simulink model "nonlinear_model_inverted_pendulum"  (R2024b)
settings: Solver=ode45  StartTime=0.0  StopTime=50  RelTol=1e-6
values from neighbouring files (symbols this model uses):
  b = 0.05    [sim_nonlinear_model_inverted_pendulum.m]
  d = r*2    (= 2)    [plotPendulo.m]    (also in sim_nonlinear_model_inverted_pendulum.m = 0.005; updatePendulo.m)
  dtheta0 = 0    [sim_nonlinear_model_inverted_pendulum.m]
  g = 9.81    [sim_nonlinear_model_inverted_pendulum.m]
  I = 0.099    [sim_nonlinear_model_inverted_pendulum.m]
  Kd1 = 0    [sim_nonlinear_model_inverted_pendulum.m]
  Kd2 = 0    [sim_nonlinear_model_inverted_pendulum.m]
  Ki1 = 0    [sim_nonlinear_model_inverted_pendulum.m]
  Ki2 = 0    [sim_nonlinear_model_inverted_pendulum.m]
  Kp1 = 0    [sim_nonlinear_model_inverted_pendulum.m]
  Kp2 = 0    [sim_nonlinear_model_inverted_pendulum.m]
  l = 40    [plotPendulo.m]    (also in sim_nonlinear_model_inverted_pendulum.m = 0.4; updatePendulo.m)
  M = 2.4    [sim_nonlinear_model_inverted_pendulum.m]
  m = 0.23    [sim_nonlinear_model_inverted_pendulum.m]    (also in unwrap.m = length(p))
  N1 = 100    [sim_nonlinear_model_inverted_pendulum.m]
  N2 = 100    [sim_nonlinear_model_inverted_pendulum.m]
  theta0 = deg2rad(5)    [sim_nonlinear_model_inverted_pendulum.m]
  theta_ref = 0    [sim_nonlinear_model_inverted_pendulum.m]
  v0 = 0    [sim_nonlinear_model_inverted_pendulum.m]
  x0 = 0.2    [sim_nonlinear_model_inverted_pendulum.m]
  x_ref = 0    [sim_nonlinear_model_inverted_pendulum.m]
undefined symbols (not defined in the file or in its folder): magnitude
libraries: slpidlib x2
settings Model: Creator=engma  LastModifiedBy=engma
settings DebuggingCC: AlgebraicLoopMsg=none

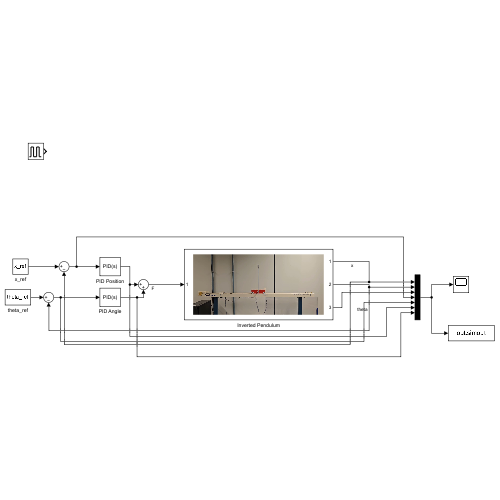
[thumbnail: Simulink's stored preview of the top-level diagram]
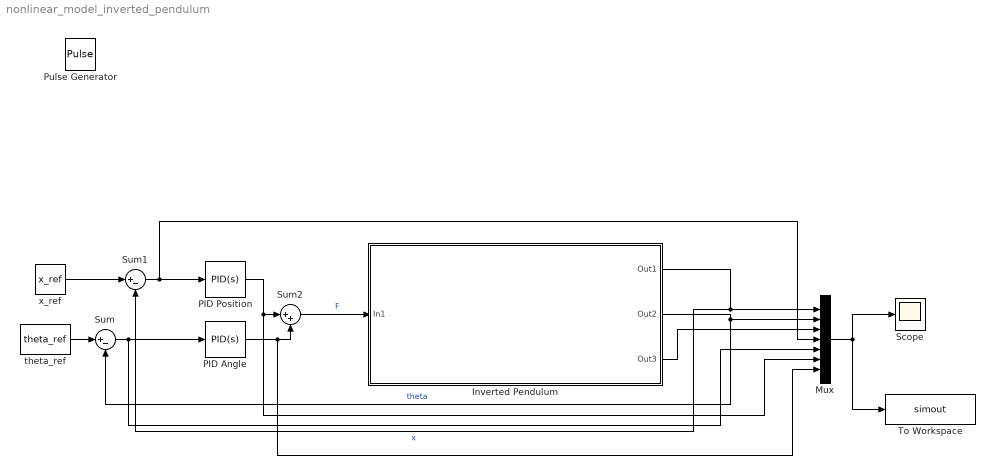
== system nonlinear_model_inverted_pendulum ==
  Inverted Pendulum : Subsystem
      mask Display: image('inverted_pendulum.jpg', [10,10,10,10,100,100]);
  Mux : Mux  Inputs=7
  PID Angle : slpidlib/PID Controller  Controller=PID  Form=Parallel  TimeDomain=Continuous-time  UseExternalTs=off  SampleTime=-1  IntegratorMethod=Forward Euler  FilterMethod=Forward Euler  ControllerParametersSource=internal  P=Kp2  I=Ki2  UseKiTs=off  D=Kd2  UseExternalDerivativeSource=off  N=N2  UseFilter=on  TunerSelectOption=Transfer Function Based (PID Tuner App)  InitialConditionSource=internal  InitialConditionForIntegrator=0  InitialConditionForFilter=0  DifferentiatorICPrevScaledInput=0  ExternalReset=none  TrackingMode=off  Kt=1  LimitOutput=off  SatLimitsSource=internal  UpperSaturationLimit=inf  LowerSaturationLimit=-inf  LinearizeAsGain=on  AntiWindupMode=none  Kb=1  LimitIntegrator=off  UpperIntegratorSaturationLimit=inf  LowerIntegratorSaturationLimit=-inf  POutMin=[]  POutMax=[]  IOutMin=[]  IOutMax=[]  DOutMin=[]  DOutMax=[]  NOutMin=[]  NOutMax=[]  SumOutMin=[]  SumOutMax=[]  SaturationOutMin=[]  SaturationOutMax=[]  PParamMin=[]  PParamMax=[]  IParamMin=[]  IParamMax=[]  DParamMin=[]  DParamMax=[]  NParamMin=[]  NParamMax=[]  KbParamMin=[]  KbParamMax=[]  KtParamMin=[]  KtParamMax=[]  KbOutMin=[]  KbOutMax=[]  KtOutMin=[]  KtOutMax=[]  IntegratorOutMin=[]  IntegratorOutMax=[]  FilterOutMin=[]  FilterOutMax=[]  SumI1OutMin=[]  SumI1OutMax=[]  SumI2OutMin=[]  SumI2OutMax=[]  SumI3OutMin=[]  SumI3OutMax=[]  SumI4OutMin=[]  SumI4OutMax=[]  SumDOutMin=[]  SumDOutMax=[]  DifferentiatorOutMin=[]  DifferentiatorOutMax=[]  FilterDiffOutCoefMin=[]  FilterDiffOutCoefMax=[]  ReciprocalOutMin=[]  ReciprocalOutMax=[]  SumDenOutMin=[]  SumDenOutMax=[]  SumNumOutMin=[]  SumNumOutMax=[]  DivideOutMin=[]  DivideOutMax=[]  UdiffTsProdOutMin=[]  UdiffTsProdOutMax=[]  NTsProdOutMin=[]  NTsProdOutMax=[]  UintegralTsProdOutMin=[]  UintegralTsProdOutMax=[]  UngainTsProdOutMin=[]  UngainTsProdOutMax=[]  ClampingZeroOutDataTypeStr=Inherit: Inherit via back propagation  ClampingZeroOutMin=[]  ClampingZeroOutMax=[]  FilterDenConstantOutDataTypeStr=Inherit: Inherit via back propagation  FilterDenConstantOutMin=[]  FilterDenConstantOutMax=[]  PCopyOutDataTypeStr=Inherit: Inherit via back propagation  PCopyOutMin=[]  PCopyOutMax=[]  NCopyOutDataTypeStr=Inherit: Inherit via back propagation  NCopyOutMin=[]  NCopyOutMax=[]  IntegratorContinuousStateAttributes=''  IntegratorStateMustResolveToSignalObject=off  IntegratorRTWStateStorageClass=Auto  FilterContinuousStateAttributes=''  FilterStateMustResolveToSignalObject=off  FilterRTWStateStorageClass=Auto  ParallelPVariant=InternalParameters  IdealPVariant=Disabled  IVariant=InternalParameters  DVariant=InternalParameters  IntegratorVariant=Continuous  SatVariant=Disabled  AWVariant=Passthrough  PCopyVariant=Disabled  TRVariant=Disabled  FdbkBlocksVariant=Forward  IdealPFdbkVariant=Disabled  SatFdbkVariant=Disabled  DerivativeFilterVariant=ContFilter  NVariant=InternalParameters  NCopyVariant=Disabled  FilterICVariant=InternalICsFilter  IntegratorICVariant=InternalICs  ExternalResetVariant=Disabled  TRSumVariant=Passthrough  SumFdbkVariant=Disabled  SumVariant=Sum_PID  TsampFilterVariant=InternalTs  TsampNgainVariant=Passthrough  TsampIntegralVariant=Disabled_SignalSpec  ExternalSaturationOutDataTypeStr=Inherit: Same as second input  DerivativeSourceVariant=ErrorSignal  PreIntVariant=InternalPreInt
  PID Position : slpidlib/PID Controller  Controller=PID  Form=Parallel  TimeDomain=Continuous-time  UseExternalTs=off  SampleTime=-1  IntegratorMethod=Forward Euler  FilterMethod=Forward Euler  ControllerParametersSource=internal  P=Kp1  I=Ki1  UseKiTs=off  D=Kd1  UseExternalDerivativeSource=off  N=N1  UseFilter=on  TunerSelectOption=Transfer Function Based (PID Tuner App)  InitialConditionSource=internal  InitialConditionForIntegrator=0  InitialConditionForFilter=0  DifferentiatorICPrevScaledInput=0  ExternalReset=none  TrackingMode=off  Kt=1  LimitOutput=off  SatLimitsSource=internal  UpperSaturationLimit=inf  LowerSaturationLimit=-inf  LinearizeAsGain=on  AntiWindupMode=none  Kb=1  LimitIntegrator=off  UpperIntegratorSaturationLimit=inf  LowerIntegratorSaturationLimit=-inf  POutMin=[]  POutMax=[]  IOutMin=[]  IOutMax=[]  DOutMin=[]  DOutMax=[]  NOutMin=[]  NOutMax=[]  SumOutMin=[]  SumOutMax=[]  SaturationOutMin=[]  SaturationOutMax=[]  PParamMin=[]  PParamMax=[]  IParamMin=[]  IParamMax=[]  DParamMin=[]  DParamMax=[]  NParamMin=[]  NParamMax=[]  KbParamMin=[]  KbParamMax=[]  KtParamMin=[]  KtParamMax=[]  KbOutMin=[]  KbOutMax=[]  KtOutMin=[]  KtOutMax=[]  IntegratorOutMin=[]  IntegratorOutMax=[]  FilterOutMin=[]  FilterOutMax=[]  SumI1OutMin=[]  SumI1OutMax=[]  SumI2OutMin=[]  SumI2OutMax=[]  SumI3OutMin=[]  SumI3OutMax=[]  SumI4OutMin=[]  SumI4OutMax=[]  SumDOutMin=[]  SumDOutMax=[]  DifferentiatorOutMin=[]  DifferentiatorOutMax=[]  FilterDiffOutCoefMin=[]  FilterDiffOutCoefMax=[]  ReciprocalOutMin=[]  ReciprocalOutMax=[]  SumDenOutMin=[]  SumDenOutMax=[]  SumNumOutMin=[]  SumNumOutMax=[]  DivideOutMin=[]  DivideOutMax=[]  UdiffTsProdOutMin=[]  UdiffTsProdOutMax=[]  NTsProdOutMin=[]  NTsProdOutMax=[]  UintegralTsProdOutMin=[]  UintegralTsProdOutMax=[]  UngainTsProdOutMin=[]  UngainTsProdOutMax=[]  ClampingZeroOutDataTypeStr=Inherit: Inherit via back propagation  ClampingZeroOutMin=[]  ClampingZeroOutMax=[]  FilterDenConstantOutDataTypeStr=Inherit: Inherit via back propagation  FilterDenConstantOutMin=[]  FilterDenConstantOutMax=[]  PCopyOutDataTypeStr=Inherit: Inherit via back propagation  PCopyOutMin=[]  PCopyOutMax=[]  NCopyOutDataTypeStr=Inherit: Inherit via back propagation  NCopyOutMin=[]  NCopyOutMax=[]  IntegratorContinuousStateAttributes=''  IntegratorStateMustResolveToSignalObject=off  IntegratorRTWStateStorageClass=Auto  FilterContinuousStateAttributes=''  FilterStateMustResolveToSignalObject=off  FilterRTWStateStorageClass=Auto  ParallelPVariant=InternalParameters  IdealPVariant=Disabled  IVariant=InternalParameters  DVariant=InternalParameters  IntegratorVariant=Continuous  SatVariant=Disabled  AWVariant=Passthrough  PCopyVariant=Disabled  TRVariant=Disabled  FdbkBlocksVariant=Forward  IdealPFdbkVariant=Disabled  SatFdbkVariant=Disabled  DerivativeFilterVariant=ContFilter  NVariant=InternalParameters  NCopyVariant=Disabled  FilterICVariant=InternalICsFilter  IntegratorICVariant=InternalICs  ExternalResetVariant=Disabled  TRSumVariant=Passthrough  SumFdbkVariant=Disabled  SumVariant=Sum_PID  TsampFilterVariant=InternalTs  TsampNgainVariant=Passthrough  TsampIntegralVariant=Disabled_SignalSpec  ExternalSaturationOutDataTypeStr=Inherit: Same as second input  DerivativeSourceVariant=ErrorSignal  PreIntVariant=InternalPreInt
  Pulse Generator : DiscretePulseGenerator  PulseType=Time based  Period=100  PulseWidth=5
  Scope : Scope
  Sum : Sum  Inputs=|+-
  Sum1 : Sum  Inputs=|+-
  Sum2 : Sum  Inputs=|++
  To Workspace : ToWorkspace  VariableName=simout  SaveFormat=Structure With Time  SampleTime=-1
  theta_ref : Constant  Value=theta_ref
  x_ref : Constant  Value=x_ref
  wires:
  Inverted Pendulum/1(Out1) -> Mux/1, Sum1/2  "x"
  Inverted Pendulum/2(Out2) -> Sum/2, Mux/2  "theta"
  Mux/1 -> Scope/1, To Workspace/1
  theta_ref/1 -> Sum/1
  x_ref/1 -> Sum1/1
  Sum/1 -> Mux/5, PID Angle/1
  Sum2/1 -> Inverted Pendulum/1(In1)  "F"
  Inverted Pendulum/3(Out3) -> Mux/3
  Sum1/1 -> PID Position/1, Mux/4
  PID Angle/1 -> Mux/7, Sum2/2
  PID Position/1 -> Mux/6, Sum2/1

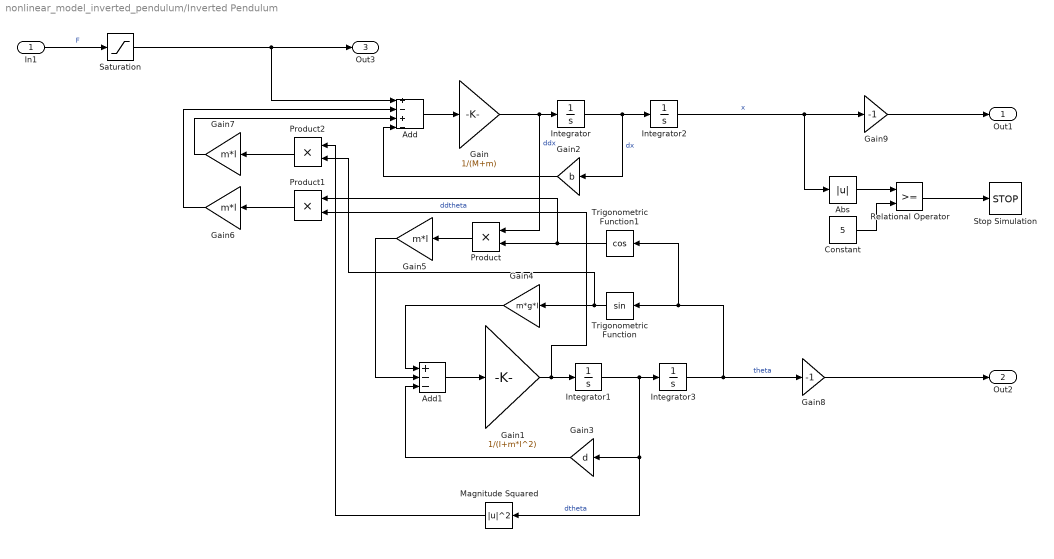
== system nonlinear_model_inverted_pendulum/Inverted Pendulum ==
  In1 : Inport
  Abs : Abs  SaturateOnIntegerOverflow=off
  Add : Sum  Inputs=+-+-
  Add1 : Sum  Inputs=+--
  Constant : Constant  Value=5
  Gain : Gain  Gain=1/(M+m)
  Gain1 : Gain  Gain=1/(I+m*l^2)
  Gain2 : Gain  Gain=b
  Gain3 : Gain  Gain=d
  Gain4 : Gain  Gain=m*g*l
  Gain5 : Gain  Gain=m*l
  Gain6 : Gain  Gain=m*l
  Gain7 : Gain  Gain=m*l
  Gain8 : Gain  Gain=-1
  Gain9 : Gain  Gain=-1
  Integrator : Integrator  InitialCondition=v0
  Integrator1 : Integrator  InitialCondition=dtheta0
  Integrator2 : Integrator  InitialCondition=x0
  Integrator3 : Integrator  InitialCondition=-theta0
  Magnitude Squared : Math  Operator=magnitude^2
  Product : Product
  Product1 : Product
  Product2 : Product
  Relational Operator : RelationalOperator  OutDataTypeStr=boolean  RndMeth=Simplest  InputSameDT=off
  Saturation : Saturate  UpperLimit=20  LowerLimit=-20
  Stop Simulation : Stop
  Trigonometric Function : Trigonometry
  Trigonometric Function1 : Trigonometry  Operator=cos
  Out1 : Outport
  Out2 : Outport  Port=2
  Out3 : Outport  Port=3
  wires:
  Gain6/1 -> Add/2
  Gain1/1 -> Product1/2, Integrator1/1  "ddtheta"
  Integrator3/1 -> Gain8/1, Trigonometric Function1/1, Trigonometric Function/1  "theta"
  Trigonometric Function1/1 -> Product1/1, Product/2
  Product/1 -> Gain5/1
  Magnitude Squared/1 -> Product2/1
  Gain/1 -> Integrator/1, Product/1  "ddx"
  Add/1 -> Gain/1
  Integrator/1 -> Gain2/1, Integrator2/1  "dx"
  Trigonometric Function/1 -> Product2/2, Gain4/1
  Gain2/1 -> Add/4
  Integrator1/1 -> Magnitude Squared/1, Gain3/1, Integrator3/1  "dtheta"
  Add1/1 -> Gain1/1
  Product1/1 -> Gain6/1
  Product2/1 -> Gain7/1
  Gain5/1 -> Add1/2
  Gain7/1 -> Add/3
  Gain3/1 -> Add1/3
  Gain4/1 -> Add1/1
  Integrator2/1 -> Gain9/1, Abs/1  "x"
  In1/1 -> Saturation/1  "F"
  Relational Operator/1 -> Stop Simulation/1
  Constant/1 -> Relational Operator/2
  Abs/1 -> Relational Operator/1
  Gain8/1 -> Out2/1
  Gain9/1 -> Out1/1
  Saturation/1 -> Add/1, Out3/1
